simulink model "InitialEstimations"  (R2018a)
settings: Solver=VariableStepAuto  StartTime=0.0  StopTime=0.2  RelTol=1e-3
settings Model: Creator=Hirsa  LastModifiedBy=Hirsa

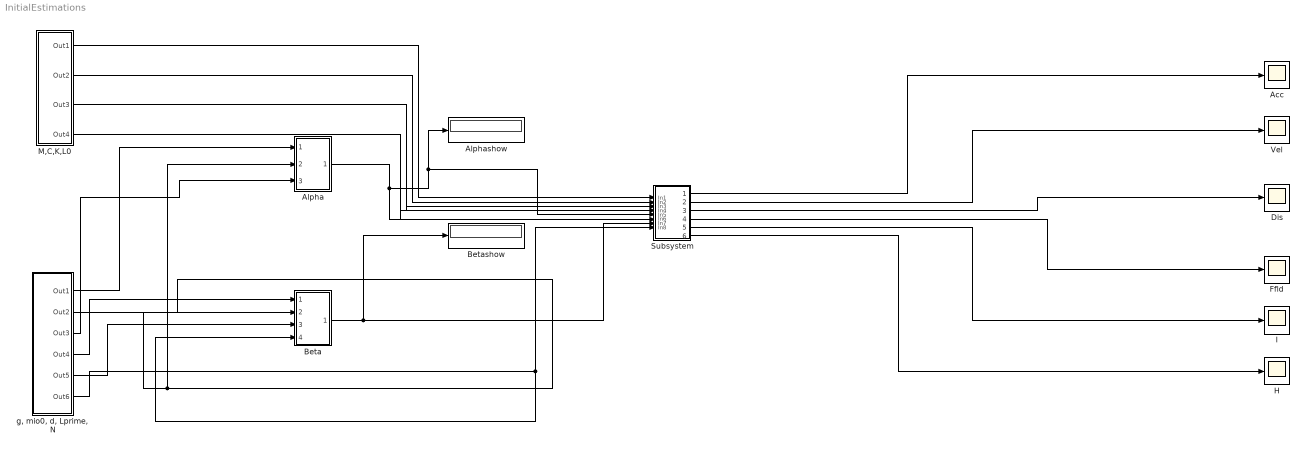
== system InitialEstimations ==
  Acc : Scope
  Alpha : Subsystem
  Alphashow : Display
  Beta : Subsystem
  Betashow : Display
  "Dis " : Scope
  Ffld : Scope
  H : Scope
  I : Scope
  M,C,K,L0 : Subsystem
  Subsystem : Subsystem
  Vel : Scope
  "g, mio0, d, Lprime, N " : Subsystem
  wires:
  Alpha/1(Out1) -> Subsystem/6(In6), Subsystem/5(In5), Alphashow/1
  Beta/1(Out1) -> Subsystem/7(In7), Betashow/1
  "g, mio0, d, Lprime, N "/2(Out2) -> Beta/2(In2), Alpha/2(In2)
  "g, mio0, d, Lprime, N "/1(Out1) -> Alpha/1(In1)
  "g, mio0, d, Lprime, N "/3(Out3) -> Alpha/3(In3)
  "g, mio0, d, Lprime, N "/4(Out4) -> Beta/1(In1)
  "g, mio0, d, Lprime, N "/5(Out5) -> Beta/3(In3)
  "g, mio0, d, Lprime, N "/6(Out6) -> Subsystem/8(In8), Beta/4(In4)
  M,C,K,L0/1(Out1) -> Subsystem/1(In1)
  M,C,K,L0/2(Out2) -> Subsystem/2(In2)
  M,C,K,L0/3(Out3) -> Subsystem/3(In3)
  M,C,K,L0/4(Out4) -> Subsystem/4(In4)
  Subsystem/1(Out1) -> Acc/1
  Subsystem/2(Out2) -> Vel/1
  Subsystem/3(Out3) -> "Dis "/1
  Subsystem/4(Out4) -> Ffld/1
  Subsystem/5(Out5) -> I/1
  Subsystem/6(Out6) -> H/1

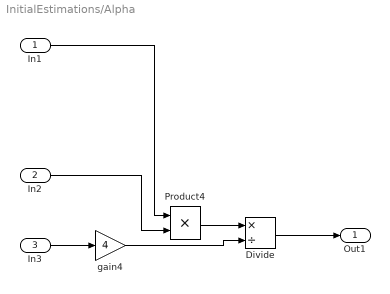
== system InitialEstimations/Alpha ==
  In1 : Inport
  In2 : Inport  Port=2
  In3 : Inport  Port=3
  Divide : Product  Inputs=*/
  Product4 : Product
  "gain4 " : Gain  Gain=4
  Out1 : Outport
  wires:
  Product4/1 -> Divide/1
  Divide/1 -> Out1/1
  In2/1 -> Product4/2
  "gain4 "/1 -> Divide/2
  In3/1 -> "gain4 "/1
  In1/1 -> Product4/1

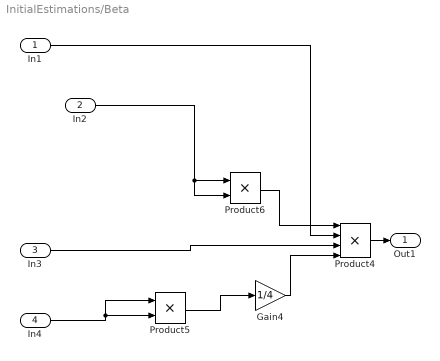
== system InitialEstimations/Beta ==
  In1 : Inport
  In2 : Inport  Port=2
  In3 : Inport  Port=3
  In4 : Inport  Port=4
  Gain4 : Gain  Gain=1/4
  Product4 : Product  Inputs=4
  Product5 : Product
  Product6 : Product
  Out1 : Outport
  wires:
  Product6/1 -> Product4/1
  In4/1 -> Product5/2, Product5/1
  In1/1 -> Product4/2
  Product5/1 -> Gain4/1
  In3/1 -> Product4/3
  Gain4/1 -> Product4/4
  In2/1 -> Product6/2, Product6/1
  Product4/1 -> Out1/1

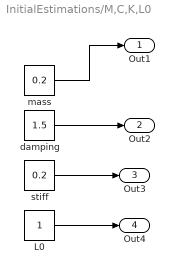
== system InitialEstimations/M,C,K,L0 ==
  L0 : Constant
  damping : Constant  Value=1.5
  mass : Constant  Value=0.2
  stiff : Constant  Value=0.2
  Out1 : Outport
  Out2 : Outport  Port=2
  Out3 : Outport  Port=3
  Out4 : Outport  Port=4
  wires:
  damping/1 -> Out2/1
  L0/1 -> Out4/1
  stiff/1 -> Out3/1
  mass/1 -> Out1/1

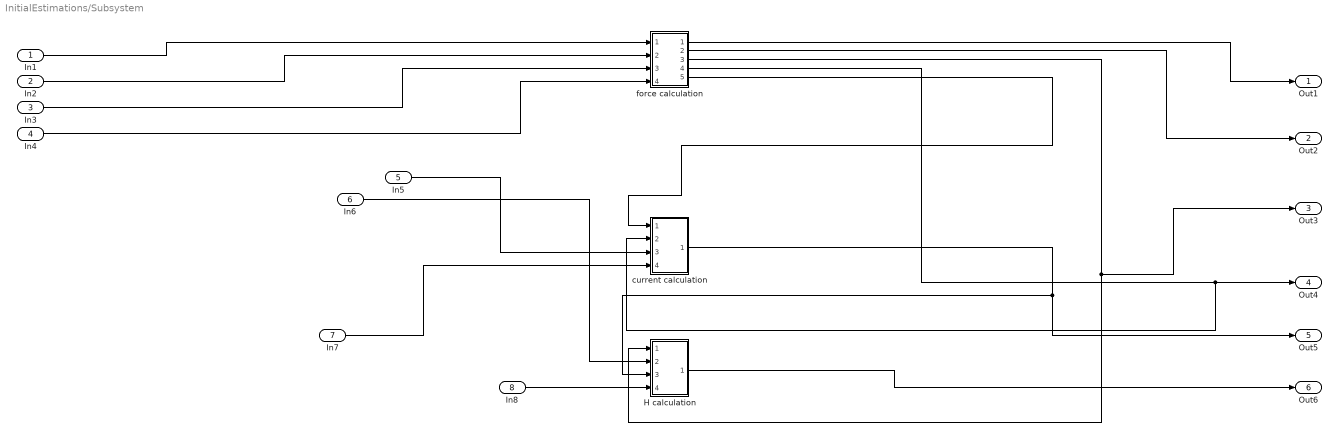
== system InitialEstimations/Subsystem ==
  In1 : Inport
  In2 : Inport  Port=2
  In3 : Inport  Port=3
  In4 : Inport  Port=4
  In5 : Inport  Port=5
  In6 : Inport  Port=6
  In7 : Inport  Port=7
  In8 : Inport  Port=8
  "H calculation " : Subsystem
  current calculation : Subsystem
  force calculation : Subsystem
  Out1 : Outport
  Out2 : Outport  Port=2
  Out3 : Outport  Port=3
  Out4 : Outport  Port=4
  Out5 : Outport  Port=5
  Out6 : Outport  Port=6
  wires:
  current calculation/1(Out1) -> Out5/1, "H calculation "/3(In3)
  In5/1 -> current calculation/3(In3)
  force calculation/3(Out3) -> Out3/1, "H calculation "/1(In1)
  In7/1 -> current calculation/4(In4)
  In1/1 -> force calculation/1(In1)
  force calculation/2(Out2) -> Out2/1
  force calculation/5(Out5) -> current calculation/1(In1)
  force calculation/4(Out4) -> Out4/1, current calculation/2(In2)
  In6/1 -> "H calculation "/2(In2)
  In2/1 -> force calculation/2(In2)
  force calculation/1(Out1) -> Out1/1
  In8/1 -> "H calculation "/4(In4)
  In4/1 -> force calculation/4(In4)
  "H calculation "/1(Out1) -> Out6/1
  In3/1 -> force calculation/3(In3)

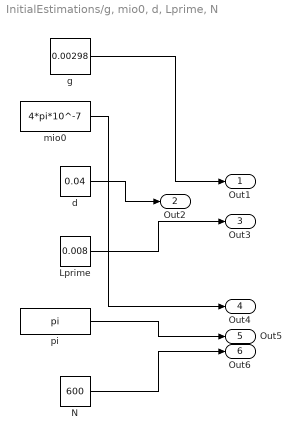
== system InitialEstimations/g, mio0, d, Lprime, N  ==
  Lprime : Constant  Value=0.008
  N : Constant  Value=600
  d : Constant  Value=0.04
  g : Constant  Value=0.00298
  mio0 : Constant  Value=4*pi*10^-7
  pi : Constant  Value=pi
  Out1 : Outport
  Out2 : Outport  Port=2
  Out3 : Outport  Port=3
  Out4 : Outport  Port=4
  Out5 : Outport  Port=5
  Out6 : Outport  Port=6
  wires:
  mio0/1 -> Out4/1
  Lprime/1 -> Out3/1
  N/1 -> Out6/1
  g/1 -> Out1/1
  d/1 -> Out2/1
  pi/1 -> Out5/1

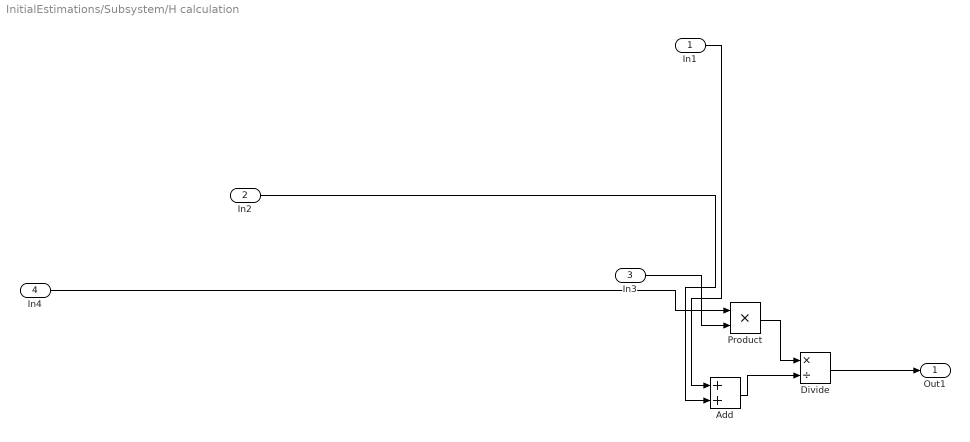
== system InitialEstimations/Subsystem/H calculation  ==
  In1 : Inport
  In2 : Inport  Port=2
  In3 : Inport  Port=3
  In4 : Inport  Port=4
  Add : Sum
  Divide : Product  Inputs=*/
  Product : Product
  Out1 : Outport
  wires:
  Add/1 -> Divide/2
  Divide/1 -> Out1/1
  In1/1 -> Add/1
  Product/1 -> Divide/1
  In4/1 -> Product/1
  In3/1 -> Product/2
  In2/1 -> Add/2

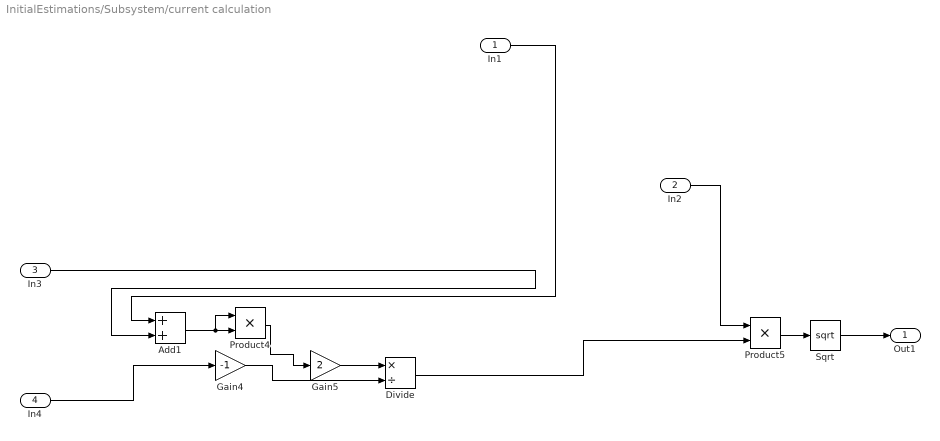
== system InitialEstimations/Subsystem/current calculation ==
  In1 : Inport
  In2 : Inport  Port=2
  In3 : Inport  Port=3
  In4 : Inport  Port=4
  Add1 : Sum
  Divide : Product  Inputs=*/
  Gain4 : Gain  Gain=-1
  Gain5 : Gain  Gain=2
  Product4 : Product
  Product5 : Product
  Sqrt : Sqrt  SaturateOnIntegerOverflow=on
  Out1 : Outport
  wires:
  Gain4/1 -> Divide/2
  Divide/1 -> Product5/2
  In1/1 -> Add1/1
  Gain5/1 -> Divide/1
  In4/1 -> Gain4/1
  Add1/1 -> Product4/1, Product4/2
  Product5/1 -> Sqrt/1
  Product4/1 -> Gain5/1
  In3/1 -> Add1/2
  Sqrt/1 -> Out1/1
  In2/1 -> Product5/1

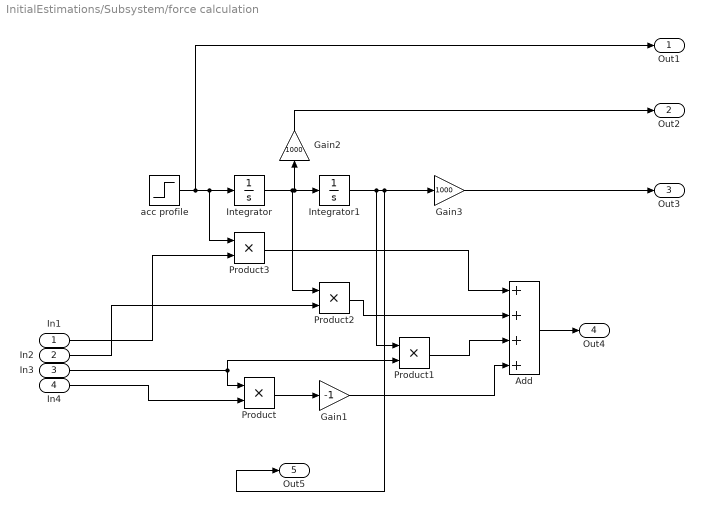
== system InitialEstimations/Subsystem/force calculation ==
  In1 : Inport
  In2 : Inport  Port=2
  In3 : Inport  Port=3
  In4 : Inport  Port=4
  Add : Sum  Inputs=++++
  Gain1 : Gain  Gain=-1
  Gain2 : Gain  Gain=1000
  Gain3 : Gain  Gain=1000
  Integrator : Integrator
  Integrator1 : Integrator  InitialCondition=0.01
  Product{,1..3} (4 alike) : Product
  acc profile : Step  Time=0.1  Before=-1  SampleTime=0
  Out1 : Outport
  Out2 : Outport  Port=2
  Out3 : Outport  Port=3
  Out4 : Outport  Port=4
  Out5 : Outport  Port=5
  wires:
  In3/1 -> Product/1, Product1/2
  Gain1/1 -> Add/4
  Gain2/1 -> Out2/1
  In4/1 -> Product/2
  acc profile/1 -> Out1/1, Product3/1, Integrator/1
  Integrator1/1 -> Product1/1, Out5/1, Gain3/1
  Product3/1 -> Add/1
  Product2/1 -> Add/2
  In1/1 -> Product3/2
  Integrator/1 -> Gain2/1, Integrator1/1, Product2/1
  Add/1 -> Out4/1
  Product/1 -> Gain1/1
  Product1/1 -> Add/3
  Gain3/1 -> Out3/1
  In2/1 -> Product2/2
